simulink model "nonlinearAirframe"  (R2019a)
settings: Solver=ode3  StartTime=0  StopTime=10.0  FixedStep=Ts  RelTol=1e-3  EnableMultiTasking=on
undefined symbols (not defined in the file): Earth, init, Vehicle, WGS84
libraries: shared6dof x1, aerolibtransform2 x1
settings Model: ExtModeTrigDuration=80  Creator=The MathWorks, Inc.  LastModifiedBy=yahyaaba
settings DataIOCC: LimitDataPoints=on  SaveFormat=Array  SaveOutput=off  SignalLogging=off  DSMLogging=off  SaveTime=off  ReturnWorkspaceOutputs=off
settings OptimizationCC: BlockReduction=off  EnhancedBackFolding=on  PassReuseOutputArgsAs=Individual arguments  MaxStackSize=64  OptimizeBlockOrder=speed  DifferentSizesBufferReuse=on  OptimizationCustomize=off
settings DebuggingCC: AlgebraicLoopMsg=none  ParameterPrecisionLossMsg=none  ParameterTunabilityLossMsg=error  UnconnectedInputMsg=none  UnconnectedOutputMsg=none  UnconnectedLineMsg=none  AllowSymbolicDim=off  SFUnexpectedBacktrackingDiag=warning  SFNoUnconditionalDefaultTransitionDiag=warning  SFExecutionAtInitializationDiag=none  ArithmeticOperatorsInVariantConditions=warning
settings HardwareCC: ProdBitPerPointer=32  ProdBitPerSizeT=32  ProdBitPerPtrDiffT=32  ProdLargestAtomicInteger=Long  ProdWordSize=32  ProdHWDeviceType=ARM Compatible->ARM 9
settings ModelReferenceCC: PropagateSignalLabelsOutOfModel=off
settings SFSimCC: SimUseLocalCustomCode=off  MATLABDynamicMemAlloc=off
settings RTWCC: SystemTargetFile=ert.tlc  HardwareBoard=PARROT Mambo  TLCOptions=-aInlineSetEventsForThisBaseRateFcn=TLC_FALSE -aSuppressMultiTaskScheduler=TLC_FALSE -aRateBasedStepFcn=1  TemplateMakefile=ert_default_tmf  GenerateReport=on  RTWUseLocalCustomCode=off  Toolchain=Sourcery G++ Lite GNU Toolchain for Drones  IncludeHyperlinkInReport=on  LaunchReport=on  GenerateTraceInfo=on  GenerateTraceReport=on  GenerateTraceReportSl=on  GenerateTraceReportSf=on  GenerateTraceReportEml=on
settings CodeAppCC: ForceParamTrailComments=on  IgnoreCustomStorageClasses=off  MaxIdLength=63  OperatorAnnotations=on  SimulinkDataObjDesc=on  SFDataObjDesc=on  InsertBlockDesc=on
settings ERTTargetCC: SupportContinuousTime=on
settings ConfigComp: CovMetricSettings=dw  CovHtmlReporting=on  CovSaveCumulativeToWorkspaceVar=on  CovSaveSingleToWorkspaceVar=on  CovExternalEMLEnable=off  CovSFcnEnable=off

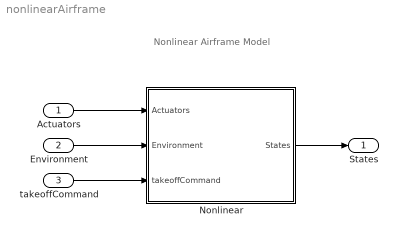
== system nonlinearAirframe ==
  note: Nonlinear Airframe Model
  Actuators : Inport  OutDataTypeStr=single  Unit=rpm  PortDimensions=[1 4]
  Environment : Inport  Port=2  OutDataTypeStr=Bus: EnvironmentBus  BusOutputAsStruct=on
  takeoffCommand : Inport  Port=3
  Nonlinear : Subsystem  TreatAsAtomicUnit=on
  States : Outport  OutDataTypeStr=Bus: StatesBus  BusOutputAsStruct=on
  wires:
  Actuators/1 -> Nonlinear/1(Actuators)
  Environment/1 -> Nonlinear/2(Environment)
  Nonlinear/1(States) -> States/1
  takeoffCommand/1 -> Nonlinear/3(takeoffCommand)

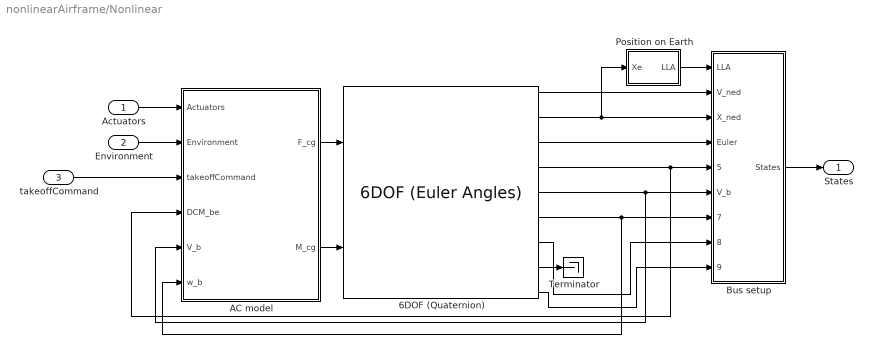
== system nonlinearAirframe/Nonlinear ==
  Actuators : Inport
  Environment : Inport  Port=2
  takeoffCommand : Inport  Port=3
  6DOF (Quaternion) : shared6dof/6DOF (Euler Angles)  units=Metric (MKS)  mtype=Fixed  rep=Euler Angles  xme_0=init.posNED  Vm_0=init.vb  eul_0=init.euler  pm_0=init.angRates  mass_0=Vehicle.Airframe.mass  mass_e=0.5  mass_f=2.0  inertia=Vehicle.Airframe.inertia  inertia_e=eye(3)  inertia_f=2*eye(3)  k_quat=Vehicle.SixDOF.quatGain  vre_flag=on  abi_flag=on  aMode=aMode  xme_statename=''  Vm_statename=''  eul_statename=''  quat_statename=''  pm_statename=''  mass_statename=''
      settings: SourceProductBaseCode=AE
  AC model : Subsystem
  Bus setup : Subsystem
  Position on Earth : Subsystem  Priority=1  TreatAsAtomicUnit=on
  Terminator : Terminator
  States : Outport
  wires:
  Actuators/1 -> AC model/1(Actuators)
  Environment/1 -> AC model/2(Environment)
  AC model/1(F_cg) -> 6DOF (Quaternion)/1
  AC model/2(M_cg) -> 6DOF (Quaternion)/2
  6DOF (Quaternion)/1 -> Bus setup/2(V_ned)
  6DOF (Quaternion)/2 -> Position on Earth/1(Xe), Bus setup/3(X_ned)
  6DOF (Quaternion)/3 -> Bus setup/4(Euler)
  6DOF (Quaternion)/6 -> AC model/6(w_b), Bus setup/7(Omega_b)
  6DOF (Quaternion)/7 -> Bus setup/8(dOmega_b)
  6DOF (Quaternion)/9 -> Bus setup/9(Accel_b)
  Bus setup/1(States) -> States/1
  Position on Earth/1(LLA) -> Bus setup/1(LLA)
  6DOF (Quaternion)/5 -> AC model/5(V_b), Bus setup/6(V_b)
  6DOF (Quaternion)/4 -> AC model/4(DCM_be), Bus setup/5(DCM_be)
  6DOF (Quaternion)/8 -> Terminator/1
  takeoffCommand/1 -> AC model/3(takeoffCommand)

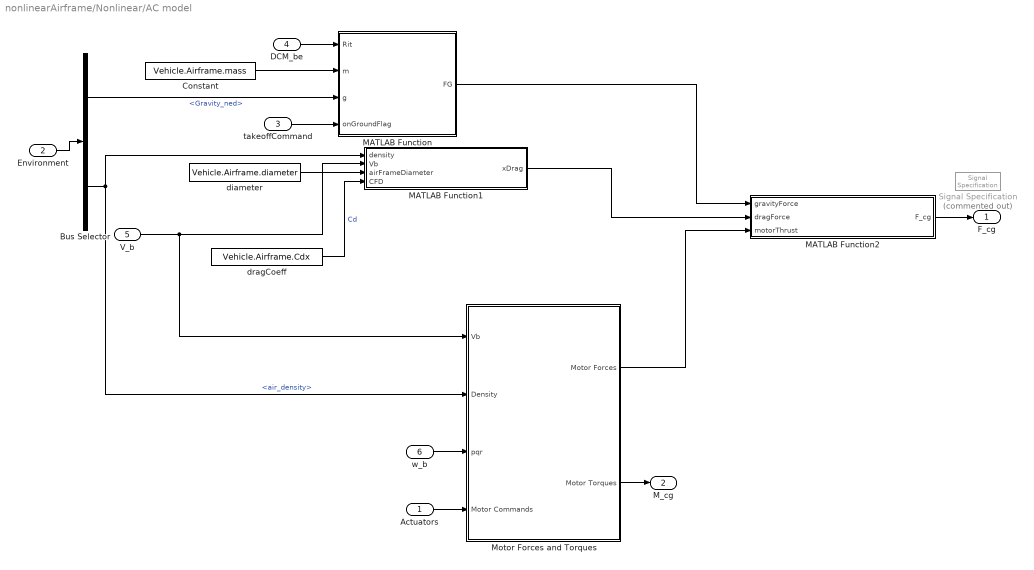
== system nonlinearAirframe/Nonlinear/AC model ==
  Actuators : Inport
  Environment : Inport  Port=2
  takeoffCommand : Inport  Port=3
  DCM_be : Inport  Port=4
  V_b : Inport  Port=5  Unit=m/s
  w_b : Inport  Port=6  Unit=rad/s
  Bus Selector : BusSelector  OutputSignals=Gravity_ned,AtmosphereBus.air_density
  Constant : Constant  Value=Vehicle.Airframe.mass
  MATLAB Function : MATLAB Function  TreatAsAtomicUnit=on
  MATLAB Function1 : MATLAB Function  TreatAsAtomicUnit=on
  MATLAB Function2 : MATLAB Function  TreatAsAtomicUnit=on
  Motor Forces and Torques : Subsystem
  Signal Specification : SignalSpecification  Commented=on  Dimensions=3
  diameter : Constant  Value=Vehicle.Airframe.diameter  SampleTime=0
  dragCoeff : Constant  Value=Vehicle.Airframe.Cdx  SampleTime=0
  F_cg : Outport  Unit=N
  M_cg : Outport  Port=2  Unit=N*m
  wires:
  Motor Forces and Torques/2(Motor Torques) -> M_cg/1
  Motor Forces and Torques/1(Motor Forces) -> MATLAB Function2/3(motorThrust)
  Bus Selector/1 -> MATLAB Function/3(g)  "<Gravity_ned>"
  Environment/1 -> Bus Selector/1
  Bus Selector/2 -> Motor Forces and Torques/2(Density), MATLAB Function1/1(density)  "<air_density>"
  DCM_be/1 -> MATLAB Function/1(Rit)
  V_b/1 -> MATLAB Function1/2(Vb), Motor Forces and Torques/1(Vb)
  MATLAB Function1/1(xDrag) -> MATLAB Function2/2(dragForce)
  Actuators/1 -> Motor Forces and Torques/4(Motor Commands)
  w_b/1 -> Motor Forces and Torques/3(pqr)
  Constant/1 -> MATLAB Function/2(m)
  MATLAB Function/1(FG) -> MATLAB Function2/1(gravityForce)
  dragCoeff/1 -> MATLAB Function1/4(CFD)  "Cd"
  diameter/1 -> MATLAB Function1/3(airFrameDiameter)
  MATLAB Function2/1(F_cg) -> F_cg/1
  takeoffCommand/1 -> MATLAB Function/4(onGroundFlag)

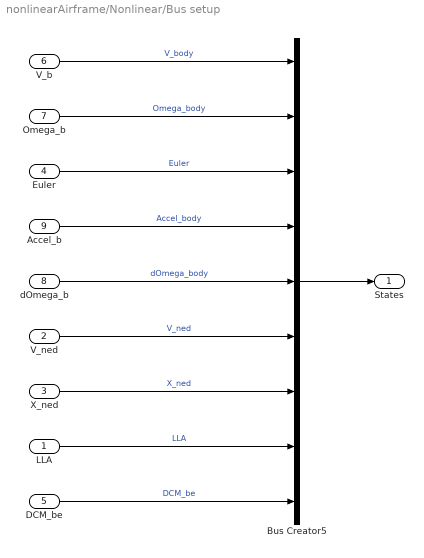
== system nonlinearAirframe/Nonlinear/Bus setup ==
  LLA : Inport  PortDimensions=3
  V_ned : Inport  Port=2  Unit=m/second  PortDimensions=3
  X_ned : Inport  Port=3  Unit=m  PortDimensions=3
  Euler : Inport  Port=4  Unit=rad  PortDimensions=3
  DCM_be : Inport  Port=5  PortDimensions=[3 3]
  V_b : Inport  Port=6  Unit=m/s  PortDimensions=3
  Omega_b : Inport  Port=7  Unit=rad/s  PortDimensions=3
  dOmega_b : Inport  Port=8  Unit=rad/s^2  PortDimensions=3
  Accel_b : Inport  Port=9  Unit=m/s^2  PortDimensions=3
  Bus Creator5 : BusCreator  Inputs=9  OutDataTypeStr=Bus: StatesBus  NonVirtualBus=on
  States : Outport
  wires:
  Bus Creator5/1 -> States/1
  V_b/1 -> Bus Creator5/1  "V_body"
  Omega_b/1 -> Bus Creator5/2  "Omega_body"
  Euler/1 -> Bus Creator5/3  "Euler"
  X_ned/1 -> Bus Creator5/7  "X_ned"
  Accel_b/1 -> Bus Creator5/4  "Accel_body"
  LLA/1 -> Bus Creator5/8  "LLA"
  dOmega_b/1 -> Bus Creator5/5  "dOmega_body"
  DCM_be/1 -> Bus Creator5/9  "DCM_be"
  V_ned/1 -> Bus Creator5/6  "V_ned"

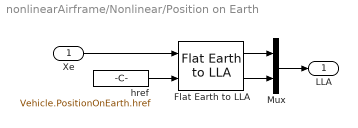
== system nonlinearAirframe/Nonlinear/Position on Earth ==
  Xe : Inport  Unit=m
  Flat Earth to LLA : aerolibtransform2/Flat Earth to LLA  units=Metric (MKS)  ptype=Earth (WGS84)  F=1/298.257223563  R=6378137  LL0=init.posLLA(1:2)  psi=Vehicle.PositionOnEarth.FlatEarthToLLA.xAxis
  Mux : Mux  Inputs=2
  href : Constant  Value=Vehicle.PositionOnEarth.href
  LLA : Outport
  wires:
  Mux/1 -> LLA/1
  Xe/1 -> Flat Earth to LLA/1
  Flat Earth to LLA/1 -> Mux/1
  Flat Earth to LLA/2 -> Mux/2
  href/1 -> Flat Earth to LLA/2

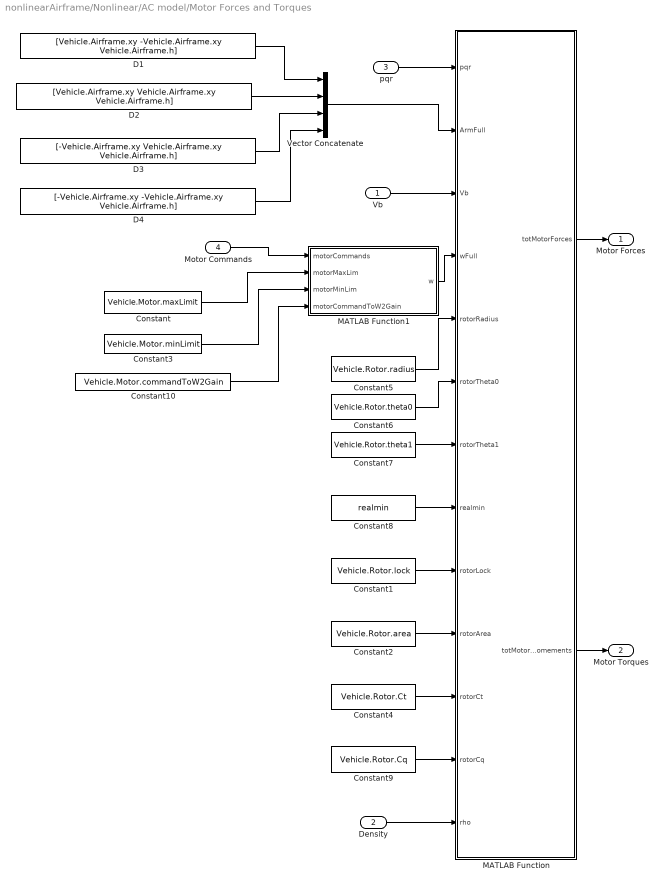
== system nonlinearAirframe/Nonlinear/AC model/Motor Forces and Torques ==
  Vb : Inport
  Density : Inport  Port=2
  pqr : Inport  Port=3
  Motor Commands : Inport  Port=4
  Constant : Constant  Value=Vehicle.Motor.maxLimit
  Constant1 : Constant  Value=Vehicle.Rotor.lock
  Constant10 : Constant  Value=Vehicle.Motor.commandToW2Gain
  Constant2 : Constant  Value=Vehicle.Rotor.area
  Constant3 : Constant  Value=Vehicle.Motor.minLimit
  Constant4 : Constant  Value=Vehicle.Rotor.Ct
  Constant5 : Constant  Value=Vehicle.Rotor.radius
  Constant6 : Constant  Value=Vehicle.Rotor.theta0
  Constant7 : Constant  Value=Vehicle.Rotor.theta1
  Constant8 : Constant  Value=realmin
  Constant9 : Constant  Value=Vehicle.Rotor.Cq
  D1 : Constant  Value=[Vehicle.Airframe.xy -Vehicle.Airframe.xy Vehicle.Airframe.h]
  D2 : Constant  Value=[Vehicle.Airframe.xy Vehicle.Airframe.xy Vehicle.Airframe.h]
  D3 : Constant  Value=[-Vehicle.Airframe.xy Vehicle.Airframe.xy Vehicle.Airframe.h]
  D4 : Constant  Value=[-Vehicle.Airframe.xy -Vehicle.Airframe.xy Vehicle.Airframe.h]
  MATLAB Function : MATLAB Function  AncestorBlock=dynamicsLibrary/Rotor Dynamics/MATLAB Function  TreatAsAtomicUnit=on
  MATLAB Function1 : MATLAB Function  TreatAsAtomicUnit=on
  Vector Concatenate : Concatenate  NumInputs=4  Mode=Multidimensional array  ConcatenateDimension=2
  Motor Forces : Outport  Unit=N
  Motor Torques : Outport  Port=2  Unit=N*m
  wires:
  MATLAB Function1/1(w) -> MATLAB Function/4(wFull)
  Constant10/1 -> MATLAB Function1/4(motorCommandToW2Gain)
  Constant/1 -> MATLAB Function1/2(motorMaxLim)
  Constant3/1 -> MATLAB Function1/3(motorMinLim)
  Density/1 -> MATLAB Function/13(rho)
  MATLAB Function/2(totMotorMomements) -> Motor Torques/1
  Motor Commands/1 -> MATLAB Function1/1(motorCommands)
  Vector Concatenate/1 -> MATLAB Function/2(ArmFull)
  MATLAB Function/1(totMotorForces) -> Motor Forces/1
  Constant6/1 -> MATLAB Function/6(rotorTheta0)
  Constant8/1 -> MATLAB Function/8(realmin)
  Constant7/1 -> MATLAB Function/7(rotorTheta1)
  Constant2/1 -> MATLAB Function/10(rotorArea)
  Constant9/1 -> MATLAB Function/12(rotorCq)
  Vb/1 -> MATLAB Function/3(Vb)
  Constant4/1 -> MATLAB Function/11(rotorCt)
  Constant5/1 -> MATLAB Function/5(rotorRadius)
  Constant1/1 -> MATLAB Function/9(rotorLock)
  pqr/1 -> MATLAB Function/1(pqr)
  D2/1 -> Vector Concatenate/2
  D3/1 -> Vector Concatenate/3
  D1/1 -> Vector Concatenate/1
  D4/1 -> Vector Concatenate/4

== matlab function nonlinearAirframe/Nonlinear/AC model/MATLAB Function1 ==
  data: density input; Vb input; xDrag output; airFrameDiameter input; CFD input
function xDrag = dragForce(density, Vb, airFrameDiameter, CFD)

q = 1/2*density*sum(Vb.^2);  % dynamic pressure : 1/2*ro*V^2

S=[airFrameDiameter*[0.25; 0.25]; airFrameDiameter];

drag=CFD*q*S;  % drag force, CFD is air frame drag coeefitien


xDrag=-sign(Vb).*drag;

== matlab function nonlinearAirframe/Nonlinear/AC model/MATLAB Function ==
  data: Rit input; FG output; m input; g input; onGroundFlag input boolean
function FG = gravityForce(Rit, m, g, onGroundFlag)

if onGroundFlag 
    FG=Rit*m*g;
else
    % when on ground, flag is 0
    FG=zeros(3,1); 
end

== matlab function nonlinearAirframe/Nonlinear/AC model/MATLAB Function2 ==
  data: gravityForce input; F_cg output; dragForce input; motorThrust input
function F_cg = appliedForce(gravityForce, dragForce, motorThrust)

F_cg = gravityForce + dragForce + motorThrust;

== matlab function nonlinearAirframe/Nonlinear/AC model/Motor Forces and Torques/MATLAB Function ==
  data: pqr input; ArmFull input; Vb input; wFull input; rotorRadius input; rotorTheta0 input; rotorTheta1 input; realmin input; rotorLock input; rotorArea input; rotorCt input; rotorCq input; rho input; totMotorForces output; totMotorMomements output
function [totMotorForces, totMotorMomements]  = rotorDynamicsFull(pqr,ArmFull, Vb, wFull, rotorRadius, rotorTheta0, rotorTheta1, realmin, rotorLock, rotorArea, rotorCt, rotorCq, rho)

motorNum=4;
motorForces=zeros(3,motorNum);
motorMomemnts=zeros(3,motorNum);

if all(wFull~=0) % all the motors have stoped
    
    for iMotor=1:motorNum
        
        w=wFull(iMotor);
        Arm=ArmFull(:,iMotor);
        
        Vr = cross(pqr, Arm)+Vb;
        
        Ic=Vr(3)/( abs(w)*rotorRadius );
        
        
        mu= real( sqrt( sum(Vr(1:2).^2) ) )/ ( abs(w)*rotorRadius );
        
        alphas=atan2(Ic,mu); % terminated
        
        
        
        if mu~=0
            tmp=[((8/3*rotorTheta0+2*rotorTheta1 )-Ic*2)/ (1./mu-0.5*mu); 0];
        else
            tmp=[((8/3*rotorTheta0+2*rotorTheta1 )-Ic*2)/ (1./realmin-0.5*mu); 0];
        end
        
        j=atan2(Vr(2), Vr(1));
        
        J=[[cos(j); sin(j)] [-sin(j); cos(j)] ];
        
        beta=J.' * tmp;
        
        tmp1=beta-( ((16/rotorLock)/abs(w)).*[pqr(2);pqr(1)] );
        
        a1s=tmp1(1);
        b1s=tmp1(2);
        
        
        Fxyz=[sin(a1s)*-cos(b1s); sin(b1s); -cos(a1s)*cos(b1s)]* w.^2 * (rotorCt*rotorRadius^2*rotorArea) * rho ;
        
        tau=cross(Arm, Fxyz);
        
        
        Mxyz=tau+[0;0; rho*abs(w)*w*(-rotorCq*rotorRadius^3*rotorArea)];
        
        motorForces(:,iMotor)=Fxyz;
        motorMomemnts(:,iMotor)=Mxyz;
    end
    
else
    % Amin
    motorForces=zeros(3,motorNum);
    motorMomemnts=zeros(3,motorNum);
end

totMotorForces=sum(motorForces,2);
totMotorMomements=sum(motorMomemnts,2);

== matlab function nonlinearAirframe/Nonlinear/AC model/Motor Forces and Torques/MATLAB Function1 ==
  data: motorCommands input; w output; motorMaxLim input; motorMinLim input; motorCommandToW2Gain input
function w = MotorsToW(motorCommands,motorMaxLim, motorMinLim, motorCommandToW2Gain)
% motor Commands to motor Speed

motorMinLim=0; % override by Amin

sat=@(A) max(min(A,motorMaxLim),motorMinLim);
signSqrt=@(A) sign(A).*sqrt(abs(A));

tmp=signSqrt( sat(motorCommands'.*[1;-1;1;-1]).*[1; -1; 1; -1] .* motorCommandToW2Gain );

w=double(tmp);
